simulink model "ups_control_non_linear_load_clean"  (R2024b)
settings: Solver=ode3  StartTime=0.0  StopTime=1  FixedStep=1e-6  MaxStep=1e-6  RelTol=1e-3
libraries: spsParallelRLCBranchLib x9, simulink x4, spsabctodq0Lib x3, eeGeneralControl x3, slpidlib x2, spsUniversalBridgeLib x2, spsGroundLib x2, spsThreePhaseVIMeasurementLib x2, spsDCVoltageSourceLib x1, spsdq0toabcLib x1, spsThreePhaseSeriesRLCBranchLib x1, sps_lib x1
settings Model: Creator=malak  LastModifiedBy=malak

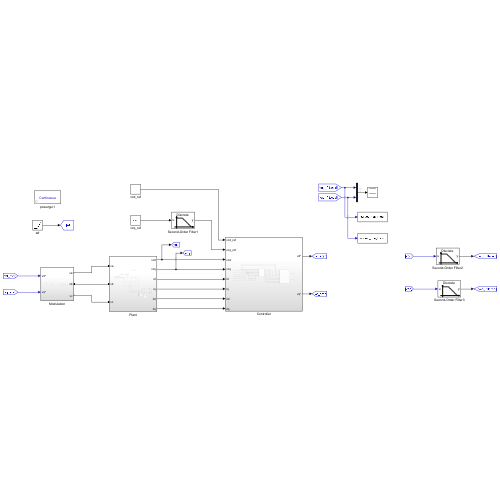
[thumbnail: Simulink's stored preview of the top-level diagram]
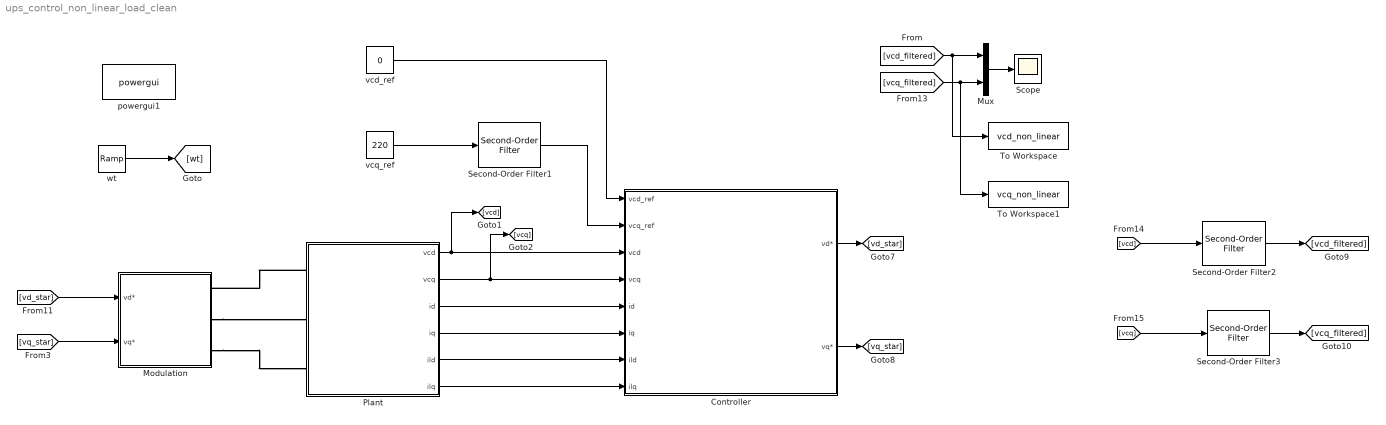
== system ups_control_non_linear_load_clean ==
  Controller : Subsystem
  Modulation : Subsystem
  Mux : Mux  Inputs=2
  Plant : Subsystem
  Scope : Scope
  Second-Order Filter1 : eeGeneralControl/Second-Order Filter  FilterType=Low-pass  fn=60  Zeta=0.707  Ts=-1  A0=0  Ph0=0  f0=0  b0=0
      settings: LibrarySourceBlock=ee_sl_lib/General Control/Second-Order Filter
  Second-Order Filter2 : eeGeneralControl/Second-Order Filter  FilterType=Low-pass  fn=60  Zeta=0.707  Ts=-1  A0=0  Ph0=0  f0=0  b0=0
      settings: LibrarySourceBlock=ee_sl_lib/General Control/Second-Order Filter
  Second-Order Filter3 : eeGeneralControl/Second-Order Filter  FilterType=Low-pass  fn=60  Zeta=0.707  Ts=-1  A0=0  Ph0=0  f0=0  b0=0
      settings: LibrarySourceBlock=ee_sl_lib/General Control/Second-Order Filter
  To Workspace : ToWorkspace  VariableName=vcd_non_linear  SaveFormat=Timeseries  SampleTime=-1
  To Workspace1 : ToWorkspace  VariableName=vcq_non_linear  SaveFormat=Timeseries  SampleTime=-1
  powergui1 : sps_lib/powergui  Priority=1  SimulationMode=Continuous  SampleTime=50e-6  frequency=60  Iterations=50  frequencyindice=0  Pbase=100e6  ErrMax=1e-4  UnitsV=kV  UnitsW=MW  buscounter=0  FunctionMessages=off  echomessages=off  EnableUseOfTLC=off  CurrentSourceSwitches=off  DisableSnubberDevices=off  DisableRonSwitches=off  DisableVfSwitches=off  DisplayEquations=off  AutomaticDiscreteSolvers=off  SolverType=Tustin/Backward Euler (TBE)  Interpol=off  ExternalGateDelay=off  methode=off  Ts=100  x0status=blocks  SPID=on  SwTol=0  HookPort=off  NonlinearTolerance=1e-4  nMaxIteration=100  ContinueOnMaxIteration=off  RestoreLinks=warning  ResistiveCurrentMeasurement=off  Frange=[0:2:500]  Ylog=off  Xlog=on  ShowGrid=off  save=off  variable=ZData  structure=0  ZoomFFT=off  StartTime=0.0  cycles=1  DisplayStyle=1  fundamental=60  FreqAxis=off  MaxFrequency=1000  frequencyindicesteady=1  RmsSteady=1  display=off
  vcd_ref : Constant  Value=0
  vcq_ref : Constant  Value=220
  wt : simulink/Sources/Ramp  slope=2*pi*60  start=0  InitialOutput=0
  wires:
  Second-Order Filter2/1 -> [vcd_filtered]
  [vcd] -> Second-Order Filter2/1
  wt/1 -> [wt]
  Second-Order Filter3/1 -> [vcq_filtered]
  Controller/1(vd*) -> [vd_star]
  [vcq_filtered] -> To Workspace1/1, Mux/2
  vcd_ref/1 -> Controller/1(vcd_ref)
  [vcq] -> Second-Order Filter3/1
  Second-Order Filter1/1 -> Controller/2(vcq_ref)
  Mux/1 -> Scope/1
  vcq_ref/1 -> Second-Order Filter1/1
  [vcd_filtered] -> To Workspace/1, Mux/1
  Controller/2(vq*) -> [vq_star]
  [vq_star] -> Modulation/2(vq*)
  [vd_star] -> Modulation/1(vd*)
  Plant/1(vcd) -> [vcd], Controller/3(vcd)
  Plant/2(vcq) -> [vcq], Controller/4(vcq)
  Plant/3(id) -> Controller/5(id)
  Plant/4(iq) -> Controller/6(iq)
  Plant/5(ild) -> Controller/7(ild)
  Plant/6(ilq) -> Controller/8(ilq)
  connections:
  Plant/LConn1 -- Modulation/RConn1
  Modulation/RConn2 -- Plant/LConn2
  Modulation/RConn3 -- Plant/LConn3

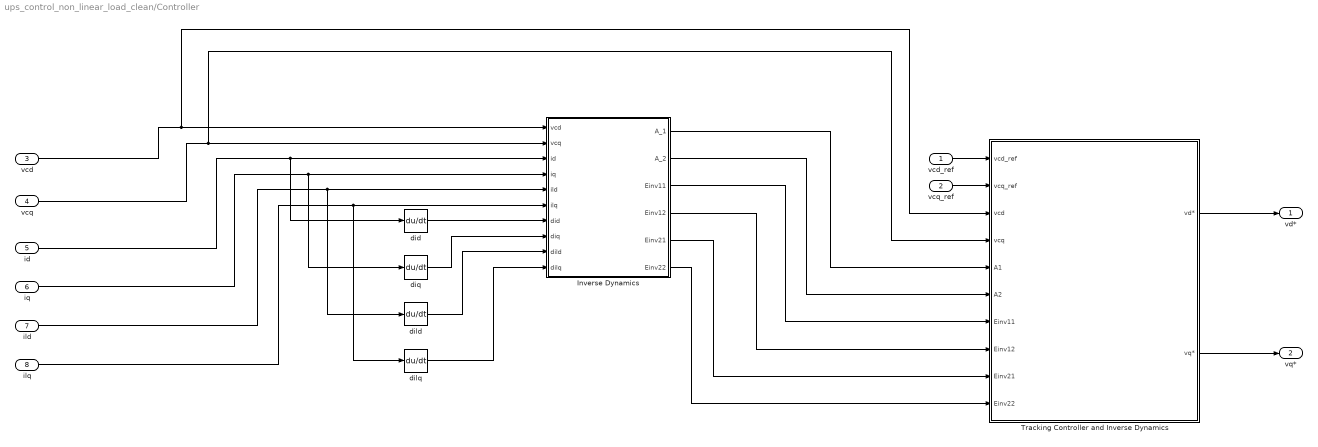
== system ups_control_non_linear_load_clean/Controller ==
  vcd_ref : Inport
  vcq_ref : Inport  Port=2
  vcd : Inport  Port=3
  vcq : Inport  Port=4
  id : Inport  Port=5
  iq : Inport  Port=6
  ild : Inport  Port=7
  ilq : Inport  Port=8
  Inverse Dynamics : MATLAB Function  TreatAsAtomicUnit=on
  Tracking Controller and Inverse Dynamics : Subsystem
  did : Derivative  CoefficientInTFapproximation=500
  dild : Derivative  CoefficientInTFapproximation=500
  dilq : Derivative  CoefficientInTFapproximation=500
  diq : Derivative  CoefficientInTFapproximation=500
  vd* : Outport
  vq* : Outport  Port=2
  wires:
  vcd/1 -> Tracking Controller and Inverse Dynamics/3(vcd), Inverse Dynamics/1(vcd)
  vcq/1 -> Tracking Controller and Inverse Dynamics/4(vcq), Inverse Dynamics/2(vcq)
  id/1 -> did/1, Inverse Dynamics/3(id)
  iq/1 -> diq/1, Inverse Dynamics/4(iq)
  ild/1 -> dild/1, Inverse Dynamics/5(ild)
  ilq/1 -> dilq/1, Inverse Dynamics/6(ilq)
  did/1 -> Inverse Dynamics/7(did)
  diq/1 -> Inverse Dynamics/8(diq)
  dild/1 -> Inverse Dynamics/9(dild)
  dilq/1 -> Inverse Dynamics/10(dilq)
  vcd_ref/1 -> Tracking Controller and Inverse Dynamics/1(vcd_ref)
  vcq_ref/1 -> Tracking Controller and Inverse Dynamics/2(vcq_ref)
  Inverse Dynamics/1(A_1) -> Tracking Controller and Inverse Dynamics/5(A1)
  Inverse Dynamics/2(A_2) -> Tracking Controller and Inverse Dynamics/6(A2)
  Inverse Dynamics/3(Einv11) -> Tracking Controller and Inverse Dynamics/7(Einv11)
  Inverse Dynamics/4(Einv12) -> Tracking Controller and Inverse Dynamics/8(Einv12)
  Inverse Dynamics/5(Einv21) -> Tracking Controller and Inverse Dynamics/9(Einv21)
  Inverse Dynamics/6(Einv22) -> Tracking Controller and Inverse Dynamics/10(Einv22)
  Tracking Controller and Inverse Dynamics/1(vd*) -> vd*/1
  Tracking Controller and Inverse Dynamics/2(vq*) -> vq*/1

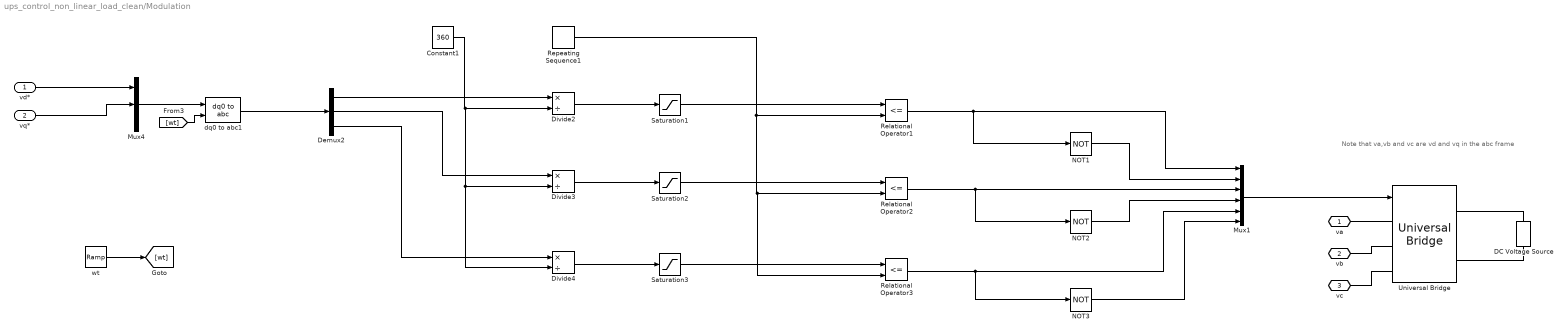
== system ups_control_non_linear_load_clean/Modulation ==
  note: Note that va,vb and vc are vd and vq in the abc frame
  vd* : Inport
  vq* : Inport  Port=2
  Constant1 : Constant  Value=360
  DC Voltage Source : spsDCVoltageSourceLib/DC Voltage Source  Amplitude=360  Measurements=None
  Demux2 : Demux  Outputs=3
  Divide2 : Product  Inputs=*/
  Divide3 : Product  Inputs=*/
  Divide4 : Product  Inputs=*/
  Mux1 : Mux  Inputs=6
  Mux4 : Mux  Inputs=3
  NOT1 : Logic  Operator=NOT  IconShape=distinctive  AllPortsSameDT=off  OutDataTypeStr=boolean
  NOT2 : Logic  Operator=NOT  IconShape=distinctive  AllPortsSameDT=off  OutDataTypeStr=boolean
  NOT3 : Logic  Operator=NOT  IconShape=distinctive  AllPortsSameDT=off  OutDataTypeStr=boolean
  Relational Operator1 : RelationalOperator  Operator=<=  OutDataTypeStr=boolean  RndMeth=Simplest  InputSameDT=off
  Relational Operator2 : RelationalOperator  Operator=<=  OutDataTypeStr=boolean  RndMeth=Simplest  InputSameDT=off
  Relational Operator3 : RelationalOperator  Operator=<=  OutDataTypeStr=boolean  RndMeth=Simplest  InputSameDT=off
  Repeating Sequence1 : simulink/Sources/Repeating Sequence  rep_seq_t=[0 5.5555555555555555555555555555556e-5 1.1111111111111111111111111111111e-4]  rep_seq_y=[-1 +1 -1]
  Saturation1 : Saturate  UpperLimit=1  LowerLimit=-1
  Saturation2 : Saturate  UpperLimit=1  LowerLimit=-1
  Saturation3 : Saturate  UpperLimit=1  LowerLimit=-1
  Universal Bridge : spsUniversalBridgeLib/Universal Bridge  Arms=3  SnubberResistance=1e5  SnubberCapacitance=inf  Device=IGBT / Diodes  Ron=1e-3  Lon=0  ForwardVoltages="[  0  0  ]"  ForwardVoltage=0  GTOparameters=[ 10e-6 , 20e-6 ]  IGBTparameters=[ 1e-6 , 2e-6 ]  Measurements=None  Measurements_2=None  converterType=Rectifier
  dq0 to abc1 : spsdq0toabcLib/dq0 to abc  Alignment=Aligned with phase A axis
  wt : simulink/Sources/Ramp  slope=2*pi*60  start=0  InitialOutput=0
  va : PMIOPort  Side=Right
  vb : PMIOPort  Port=2  Side=Right
  vc : PMIOPort  Port=3  Side=Right
  wires:
  Constant1/1 -> Divide2/2, Divide3/2, Divide4/2
  Mux4/1 -> dq0 to abc1/1
  Saturation1/1 -> Relational Operator1/1
  NOT2/1 -> Mux1/4
  Mux1/1 -> Universal Bridge/1
  vq*/1 -> Mux4/2
  Demux2/2 -> Divide3/1
  NOT3/1 -> Mux1/6
  Saturation2/1 -> Relational Operator2/1
  Relational Operator1/1 -> Mux1/1, NOT1/1
  Relational Operator3/1 -> Mux1/5, NOT3/1
  vd*/1 -> Mux4/1
  Divide2/1 -> Saturation1/1
  Repeating Sequence1/1 -> Relational Operator1/2, Relational Operator2/2, Relational Operator3/2
  Demux2/3 -> Divide4/1
  dq0 to abc1/1 -> Demux2/1
  NOT1/1 -> Mux1/2
  Divide3/1 -> Saturation2/1
  [wt] -> dq0 to abc1/2
  Saturation3/1 -> Relational Operator3/1
  Demux2/1 -> Divide2/1
  Divide4/1 -> Saturation3/1
  Relational Operator2/1 -> Mux1/3, NOT2/1
  wt/1 -> [wt]
  connections:
  Universal Bridge/LConn1 -- va/RConn1
  DC Voltage Source/LConn1 -- Universal Bridge/RConn2
  DC Voltage Source/RConn1 -- Universal Bridge/RConn1
  Universal Bridge/LConn2 -- vb/RConn1
  Universal Bridge/LConn3 -- vc/RConn1

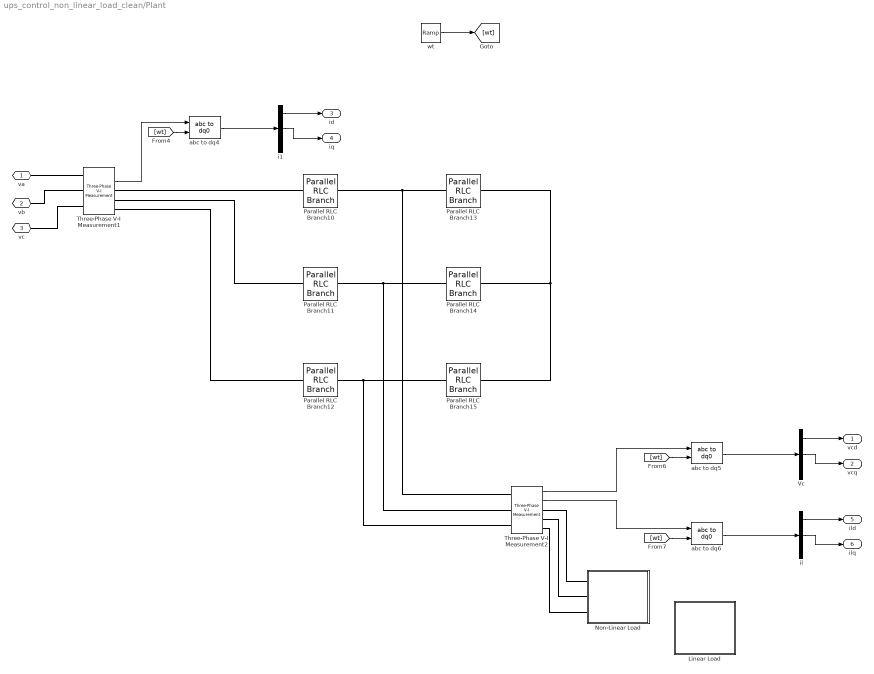
== system ups_control_non_linear_load_clean/Plant ==
  Linear Load : Subsystem
  Non-Linear Load : Subsystem
  Parallel RLC Branch10 : spsParallelRLCBranchLib/Parallel RLC Branch  LConnTagsString=a  RConnTagsString=__new0  BranchType=L  Resistance=10  Inductance=0.000800  SetiL0=off  InitialCurrent=0  Capacitance=0.001650  Setx0=off  InitialVoltage=0  Measurements=None
  Parallel RLC Branch11 : spsParallelRLCBranchLib/Parallel RLC Branch  LConnTagsString=a  RConnTagsString=__new0  BranchType=L  Resistance=10  Inductance=0.000800  SetiL0=off  InitialCurrent=0  Capacitance=0.001650  Setx0=off  InitialVoltage=0  Measurements=None
  Parallel RLC Branch12 : spsParallelRLCBranchLib/Parallel RLC Branch  LConnTagsString=a  RConnTagsString=__new0  BranchType=L  Resistance=10  Inductance=0.000800  SetiL0=off  InitialCurrent=0  Capacitance=0.001650  Setx0=off  InitialVoltage=0  Measurements=None
  Parallel RLC Branch13 : spsParallelRLCBranchLib/Parallel RLC Branch  LConnTagsString=a  RConnTagsString=__new0  BranchType=C  Resistance=10  Inductance=0.000800  SetiL0=off  InitialCurrent=0  Capacitance=0.000075  Setx0=off  InitialVoltage=0  Measurements=None
  Parallel RLC Branch14 : spsParallelRLCBranchLib/Parallel RLC Branch  LConnTagsString=a  RConnTagsString=__new0  BranchType=C  Resistance=10  Inductance=0.000800  SetiL0=off  InitialCurrent=0  Capacitance=0.000075  Setx0=off  InitialVoltage=0  Measurements=None
  Parallel RLC Branch15 : spsParallelRLCBranchLib/Parallel RLC Branch  LConnTagsString=a  RConnTagsString=__new0  BranchType=C  Resistance=10  Inductance=0.000800  SetiL0=off  InitialCurrent=0  Capacitance=0.000075  Setx0=off  InitialVoltage=0  Measurements=None
  Three-Phase V-I Measurement1 : spsThreePhaseVIMeasurementLib/Three-Phase V-I Measurement  VoltageMeasurement=phase-to-ground  SetLabelV=off  LabelV=Vabc  Vpu=off  VpuLL=off  CurrentMeasurement=yes  SetLabelI=off  LabelI=Iabc  Ipu=off  Pbase=100e6  Vbase=500e3  OutputType=Complex  PhasorSimulation=off  PSBequivalent=0
  Three-Phase V-I Measurement2 : spsThreePhaseVIMeasurementLib/Three-Phase V-I Measurement  VoltageMeasurement=phase-to-ground  SetLabelV=off  LabelV=Vabc  Vpu=off  VpuLL=off  CurrentMeasurement=yes  SetLabelI=off  LabelI=Iabc  Ipu=off  Pbase=100e6  Vbase=500e3  OutputType=Complex  PhasorSimulation=off  PSBequivalent=0
  Vc : Demux  Outputs=3
  abc to dq4 : spsabctodq0Lib/abc to dq0  Alignment=Aligned with phase A axis
  abc to dq5 : spsabctodq0Lib/abc to dq0  Alignment=Aligned with phase A axis
  abc to dq6 : spsabctodq0Lib/abc to dq0  Alignment=Aligned with phase A axis
  i1 : Demux  Outputs=3
  il : Demux  Outputs=3
  wt : simulink/Sources/Ramp  slope=2*pi*60  start=0  InitialOutput=0
  va : PMIOPort  Side=Left
  vb : PMIOPort  Port=2  Side=Left
  vc : PMIOPort  Port=3  Side=Left
  vcd : Outport
  vcq : Outport  Port=2
  id : Outport  Port=3
  iq : Outport  Port=4
  ild : Outport  Port=5
  ilq : Outport  Port=6
  wires:
  abc to dq4/1 -> i1/1
  il/1 -> ild/1
  i1/1 -> id/1
  Three-Phase V-I Measurement1/2 -> abc to dq4/1
  il/2 -> ilq/1
  i1/2 -> iq/1
  Vc/2 -> vcq/1
  [wt] -> abc to dq5/2
  Three-Phase V-I Measurement2/1 -> abc to dq5/1
  abc to dq5/1 -> Vc/1
  abc to dq6/1 -> il/1
  [wt] -> abc to dq6/2
  Vc/1 -> vcd/1
  Three-Phase V-I Measurement2/2 -> abc to dq6/1
  [wt] -> abc to dq4/2
  wt/1 -> [wt]
  connections:
  Three-Phase V-I Measurement2/LConn3 -- Parallel RLC Branch12/RConn1 -- Parallel RLC Branch15/LConn1
  Parallel RLC Branch14/RConn1 -- Parallel RLC Branch15/RConn1 -- Parallel RLC Branch13/RConn1
  Three-Phase V-I Measurement2/LConn2 -- Parallel RLC Branch14/LConn1 -- Parallel RLC Branch11/RConn1
  Three-Phase V-I Measurement2/LConn1 -- Parallel RLC Branch13/LConn1 -- Parallel RLC Branch10/RConn1
  Three-Phase V-I Measurement1/RConn3 -- Parallel RLC Branch12/LConn1
  va/RConn1 -- Three-Phase V-I Measurement1/LConn1
  Parallel RLC Branch10/LConn1 -- Three-Phase V-I Measurement1/RConn1
  Three-Phase V-I Measurement1/RConn2 -- Parallel RLC Branch11/LConn1
  vb/RConn1 -- Three-Phase V-I Measurement1/LConn2
  vc/RConn1 -- Three-Phase V-I Measurement1/LConn3
  Non-Linear Load/LConn1 -- Three-Phase V-I Measurement2/RConn1
  Non-Linear Load/LConn2 -- Three-Phase V-I Measurement2/RConn2
  Non-Linear Load/LConn3 -- Three-Phase V-I Measurement2/RConn3

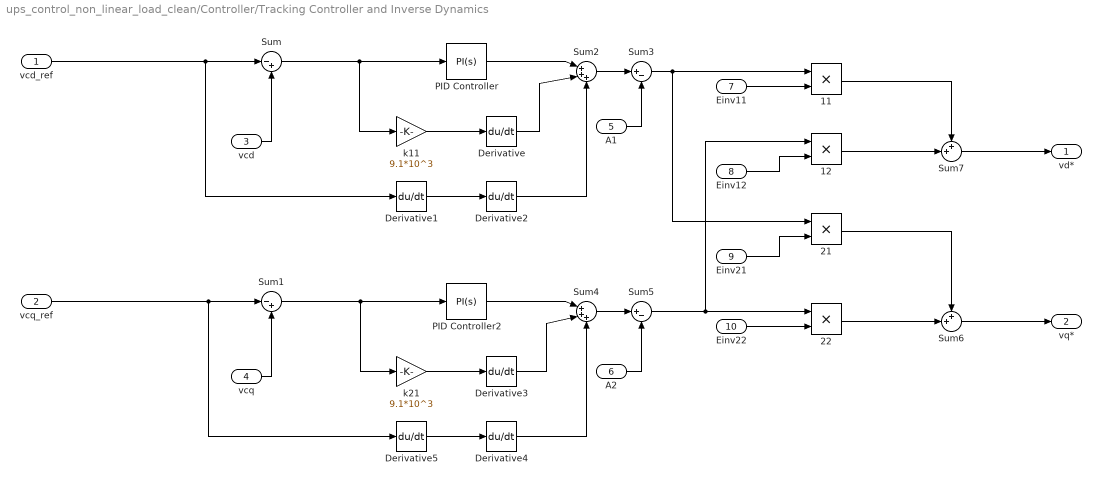
== system ups_control_non_linear_load_clean/Controller/Tracking Controller and Inverse Dynamics ==
  vcd_ref : Inport
  vcq_ref : Inport  Port=2
  vcd : Inport  Port=3
  vcq : Inport  Port=4
  A1 : Inport  Port=5
  A2 : Inport  Port=6
  Einv11 : Inport  Port=7
  Einv12 : Inport  Port=8
  Einv21 : Inport  Port=9
  Einv22 : Inport  Port=10
  {11..12,21..22} (4 alike) : Product
  Derivative{,1..5} (6 alike) : Derivative  CoefficientInTFapproximation=500
  PID Controller : slpidlib/PID Controller  Controller=PI  Form=Parallel  TimeDomain=Continuous-time  UseExternalTs=off  SampleTime=-1  IntegratorMethod=Forward Euler  FilterMethod=Forward Euler  ControllerParametersSource=internal  P=2.115*10^7  I=2.025*10^9  UseKiTs=off  D=0  UseExternalDerivativeSource=off  N=100  UseFilter=on  TunerSelectOption=Transfer Function Based (PID Tuner App)  InitialConditionSource=internal  InitialConditionForIntegrator=0  InitialConditionForFilter=0  DifferentiatorICPrevScaledInput=0  ExternalReset=none  TrackingMode=off  Kt=1  LimitOutput=off  SatLimitsSource=internal  UpperSaturationLimit=inf  LowerSaturationLimit=-inf  LinearizeAsGain=on  AntiWindupMode=none  Kb=1  LimitIntegrator=off  UpperIntegratorSaturationLimit=inf  LowerIntegratorSaturationLimit=-inf  POutMin=[]  POutMax=[]  IOutMin=[]  IOutMax=[]  DOutMin=[]  DOutMax=[]  NOutMin=[]  NOutMax=[]  SumOutMin=[]  SumOutMax=[]  SaturationOutMin=[]  SaturationOutMax=[]  PParamMin=[]  PParamMax=[]  IParamMin=[]  IParamMax=[]  DParamMin=[]  DParamMax=[]  NParamMin=[]  NParamMax=[]  KbParamMin=[]  KbParamMax=[]  KtParamMin=[]  KtParamMax=[]  KbOutMin=[]  KbOutMax=[]  KtOutMin=[]  KtOutMax=[]  IntegratorOutMin=[]  IntegratorOutMax=[]  FilterOutMin=[]  FilterOutMax=[]  SumI1OutMin=[]  SumI1OutMax=[]  SumI2OutMin=[]  SumI2OutMax=[]  SumI3OutMin=[]  SumI3OutMax=[]  SumI4OutMin=[]  SumI4OutMax=[]  SumDOutMin=[]  SumDOutMax=[]  DifferentiatorOutMin=[]  DifferentiatorOutMax=[]  FilterDiffOutCoefMin=[]  FilterDiffOutCoefMax=[]  ReciprocalOutMin=[]  ReciprocalOutMax=[]  SumDenOutMin=[]  SumDenOutMax=[]  SumNumOutMin=[]  SumNumOutMax=[]  DivideOutMin=[]  DivideOutMax=[]  UdiffTsProdOutMin=[]  UdiffTsProdOutMax=[]  NTsProdOutMin=[]  NTsProdOutMax=[]  UintegralTsProdOutMin=[]  UintegralTsProdOutMax=[]  UngainTsProdOutMin=[]  UngainTsProdOutMax=[]  ClampingZeroOutDataTypeStr=Inherit: Inherit via back propagation  ClampingZeroOutMin=[]  ClampingZeroOutMax=[]  FilterDenConstantOutDataTypeStr=Inherit: Inherit via back propagation  FilterDenConstantOutMin=[]  FilterDenConstantOutMax=[]  PCopyOutDataTypeStr=Inherit: Inherit via back propagation  PCopyOutMin=[]  PCopyOutMax=[]  NCopyOutDataTypeStr=Inherit: Inherit via back propagation  NCopyOutMin=[]  NCopyOutMax=[]  IntegratorContinuousStateAttributes=''  IntegratorStateMustResolveToSignalObject=off  IntegratorRTWStateStorageClass=Auto  FilterContinuousStateAttributes=''  FilterStateMustResolveToSignalObject=off  FilterRTWStateStorageClass=Auto  ParallelPVariant=InternalParameters  IdealPVariant=Disabled  IVariant=InternalParameters  DVariant=Disabled  IntegratorVariant=Continuous  SatVariant=Disabled  AWVariant=Passthrough  PCopyVariant=Disabled  TRVariant=Disabled  FdbkBlocksVariant=Forward  IdealPFdbkVariant=Disabled  SatFdbkVariant=Disabled  DerivativeFilterVariant=Disabled  NVariant=Disabled  NCopyVariant=Disabled_SignalSpec  FilterICVariant=Disabled  IntegratorICVariant=InternalICs  ExternalResetVariant=Disabled  TRSumVariant=Passthrough  SumFdbkVariant=Disabled  SumVariant=Sum_PI  TsampFilterVariant=InternalTs  TsampNgainVariant=Passthrough  TsampIntegralVariant=Disabled_SignalSpec  ExternalSaturationOutDataTypeStr=Inherit: Same as second input  DerivativeSourceVariant=Disabled  PreIntVariant=InternalPreInt
  PID Controller2 : slpidlib/PID Controller  Controller=PI  Form=Parallel  TimeDomain=Continuous-time  UseExternalTs=off  SampleTime=-1  IntegratorMethod=Forward Euler  FilterMethod=Forward Euler  ControllerParametersSource=internal  P=2.115*10^7  I=2.025*10^9  UseKiTs=off  D=0  UseExternalDerivativeSource=off  N=100  UseFilter=on  TunerSelectOption=Transfer Function Based (PID Tuner App)  InitialConditionSource=internal  InitialConditionForIntegrator=0  InitialConditionForFilter=0  DifferentiatorICPrevScaledInput=0  ExternalReset=none  TrackingMode=off  Kt=1  LimitOutput=off  SatLimitsSource=internal  UpperSaturationLimit=inf  LowerSaturationLimit=-inf  LinearizeAsGain=on  AntiWindupMode=none  Kb=1  LimitIntegrator=off  UpperIntegratorSaturationLimit=inf  LowerIntegratorSaturationLimit=-inf  POutMin=[]  POutMax=[]  IOutMin=[]  IOutMax=[]  DOutMin=[]  DOutMax=[]  NOutMin=[]  NOutMax=[]  SumOutMin=[]  SumOutMax=[]  SaturationOutMin=[]  SaturationOutMax=[]  PParamMin=[]  PParamMax=[]  IParamMin=[]  IParamMax=[]  DParamMin=[]  DParamMax=[]  NParamMin=[]  NParamMax=[]  KbParamMin=[]  KbParamMax=[]  KtParamMin=[]  KtParamMax=[]  KbOutMin=[]  KbOutMax=[]  KtOutMin=[]  KtOutMax=[]  IntegratorOutMin=[]  IntegratorOutMax=[]  FilterOutMin=[]  FilterOutMax=[]  SumI1OutMin=[]  SumI1OutMax=[]  SumI2OutMin=[]  SumI2OutMax=[]  SumI3OutMin=[]  SumI3OutMax=[]  SumI4OutMin=[]  SumI4OutMax=[]  SumDOutMin=[]  SumDOutMax=[]  DifferentiatorOutMin=[]  DifferentiatorOutMax=[]  FilterDiffOutCoefMin=[]  FilterDiffOutCoefMax=[]  ReciprocalOutMin=[]  ReciprocalOutMax=[]  SumDenOutMin=[]  SumDenOutMax=[]  SumNumOutMin=[]  SumNumOutMax=[]  DivideOutMin=[]  DivideOutMax=[]  UdiffTsProdOutMin=[]  UdiffTsProdOutMax=[]  NTsProdOutMin=[]  NTsProdOutMax=[]  UintegralTsProdOutMin=[]  UintegralTsProdOutMax=[]  UngainTsProdOutMin=[]  UngainTsProdOutMax=[]  ClampingZeroOutDataTypeStr=Inherit: Inherit via back propagation  ClampingZeroOutMin=[]  ClampingZeroOutMax=[]  FilterDenConstantOutDataTypeStr=Inherit: Inherit via back propagation  FilterDenConstantOutMin=[]  FilterDenConstantOutMax=[]  PCopyOutDataTypeStr=Inherit: Inherit via back propagation  PCopyOutMin=[]  PCopyOutMax=[]  NCopyOutDataTypeStr=Inherit: Inherit via back propagation  NCopyOutMin=[]  NCopyOutMax=[]  IntegratorContinuousStateAttributes=''  IntegratorStateMustResolveToSignalObject=off  IntegratorRTWStateStorageClass=Auto  FilterContinuousStateAttributes=''  FilterStateMustResolveToSignalObject=off  FilterRTWStateStorageClass=Auto  ParallelPVariant=InternalParameters  IdealPVariant=Disabled  IVariant=InternalParameters  DVariant=Disabled  IntegratorVariant=Continuous  SatVariant=Disabled  AWVariant=Passthrough  PCopyVariant=Disabled  TRVariant=Disabled  FdbkBlocksVariant=Forward  IdealPFdbkVariant=Disabled  SatFdbkVariant=Disabled  DerivativeFilterVariant=Disabled  NVariant=Disabled  NCopyVariant=Disabled_SignalSpec  FilterICVariant=Disabled  IntegratorICVariant=InternalICs  ExternalResetVariant=Disabled  TRSumVariant=Passthrough  SumFdbkVariant=Disabled  SumVariant=Sum_PI  TsampFilterVariant=InternalTs  TsampNgainVariant=Passthrough  TsampIntegralVariant=Disabled_SignalSpec  ExternalSaturationOutDataTypeStr=Inherit: Same as second input  DerivativeSourceVariant=Disabled  PreIntVariant=InternalPreInt
  Sum : Sum  Inputs=|-+
  Sum1 : Sum  Inputs=|-+
  Sum2 : Sum  Inputs=|+++
  Sum3 : Sum  Inputs=|+-
  Sum4 : Sum  Inputs=|+++
  Sum5 : Sum  Inputs=|+-
  Sum6 : Sum  Inputs=++|
  Sum7 : Sum  Inputs=++|
  k11 : Gain  Gain=9.1*10^3
  k21 : Gain  Gain=9.1*10^3
  vd* : Outport
  vq* : Outport  Port=2
  wires:
  Sum2/1 -> Sum3/1
  Sum4/1 -> Sum5/1
  Derivative/1 -> Sum2/2
  Sum1/1 -> k21/1, PID Controller2/1
  vcd_ref/1 -> Sum/1, Derivative1/1
  PID Controller2/1 -> Sum4/1
  PID Controller/1 -> Sum2/1
  22/1 -> Sum6/2
  21/1 -> Sum6/1
  11/1 -> Sum7/1
  Sum5/1 -> 12/1, 22/1
  Derivative2/1 -> Sum2/3
  12/1 -> Sum7/2
  Sum3/1 -> 11/1, 21/1
  Derivative3/1 -> Sum4/2
  Sum/1 -> k11/1, PID Controller/1
  k11/1 -> Derivative/1
  Derivative1/1 -> Derivative2/1
  vcd/1 -> Sum/2
  vcq_ref/1 -> Derivative5/1, Sum1/1
  vcq/1 -> Sum1/2
  k21/1 -> Derivative3/1
  Derivative5/1 -> Derivative4/1
  Derivative4/1 -> Sum4/3
  A1/1 -> Sum3/2
  A2/1 -> Sum5/2
  Einv11/1 -> 11/2
  Einv12/1 -> 12/2
  Einv21/1 -> 21/2
  Einv22/1 -> 22/2
  Sum6/1 -> vq*/1
  Sum7/1 -> vd*/1

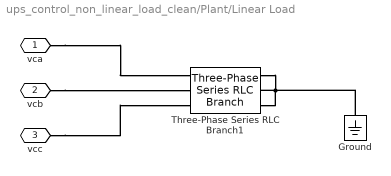
== system ups_control_non_linear_load_clean/Plant/Linear Load ==
  Ground : spsGroundLib/Ground  LConnTagsString=a
  Three-Phase Series RLC Branch1 : spsThreePhaseSeriesRLCBranchLib/Three-Phase Series RLC Branch  LConnTagsString=A|B|C  RConnTagsString=A|B|C  BranchType=RL  Resistance=10  Inductance=0.0035  Capacitance=1e-6  Measurements=None
  vca : PMIOPort  Side=Left
  vcb : PMIOPort  Port=2  Side=Left
  vcc : PMIOPort  Port=3  Side=Left
  connections:
  Ground/LConn1 -- Three-Phase Series RLC Branch1/RConn2 -- Three-Phase Series RLC Branch1/RConn3 -- Three-Phase Series RLC Branch1/RConn1
  vcb/RConn1 -- Three-Phase Series RLC Branch1/LConn2
  vcc/RConn1 -- Three-Phase Series RLC Branch1/LConn3
  vca/RConn1 -- Three-Phase Series RLC Branch1/LConn1

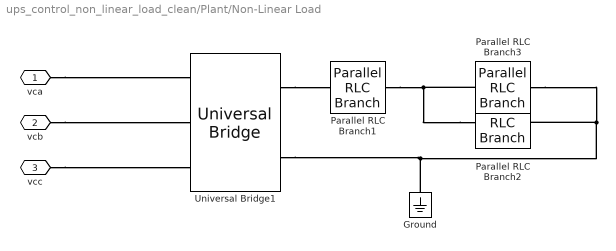
== system ups_control_non_linear_load_clean/Plant/Non-Linear Load ==
  Ground : spsGroundLib/Ground  LConnTagsString=a
  Parallel RLC Branch1 : spsParallelRLCBranchLib/Parallel RLC Branch  LConnTagsString=a  RConnTagsString=__new0  BranchType=L  Resistance=10  Inductance=0.0047  SetiL0=off  InitialCurrent=0  Capacitance=0.001650  Setx0=off  InitialVoltage=0  Measurements=None
  Parallel RLC Branch2 : spsParallelRLCBranchLib/Parallel RLC Branch  LConnTagsString=a  RConnTagsString=__new0  BranchType=R  Resistance=40  Inductance=0.000800  SetiL0=off  InitialCurrent=0  Capacitance=0.000075  Setx0=off  InitialVoltage=0  Measurements=None
  Parallel RLC Branch3 : spsParallelRLCBranchLib/Parallel RLC Branch  LConnTagsString=a  RConnTagsString=__new0  BranchType=C  Resistance=10  Inductance=0.000800  SetiL0=off  InitialCurrent=0  Capacitance=0.001650  Setx0=off  InitialVoltage=0  Measurements=None
  Universal Bridge1 : spsUniversalBridgeLib/Universal Bridge  Arms=3  SnubberResistance=1e5  SnubberCapacitance=inf  Device=Diodes  Ron=1e-3  Lon=0  ForwardVoltages="[  0  0  ]"  ForwardVoltage=0  GTOparameters=[ 10e-6 , 20e-6 ]  IGBTparameters=[ 1e-6 , 2e-6 ]  Measurements=None  Measurements_2=None  converterType=Rectifier
  vca : PMIOPort  Side=Left
  vcb : PMIOPort  Port=2  Side=Left
  vcc : PMIOPort  Port=3  Side=Left
  connections:
  vcb/RConn1 -- Universal Bridge1/LConn2
  vcc/RConn1 -- Universal Bridge1/LConn3
  vca/RConn1 -- Universal Bridge1/LConn1
  Universal Bridge1/RConn1 -- Parallel RLC Branch1/LConn1
  Parallel RLC Branch2/LConn1 -- Parallel RLC Branch3/LConn1 -- Parallel RLC Branch1/RConn1
  Parallel RLC Branch2/RConn1 -- Parallel RLC Branch3/RConn1 -- Ground/LConn1 -- Universal Bridge1/RConn2

== matlab function ups_control_non_linear_load_clean/Controller/Inverse Dynamics ==
  data: vcd input; vcq input; A_1 output; A_2 output; id input; iq input; ild input; ilq input; did input; diq input; dild input; Einv11 output; dilq input; Einv12 output; Einv21 output; Einv22 output
function [A_1,A_2,Einv11,Einv12,Einv21,Einv22] = Inverse_Dynamics(vcd,vcq,id,iq,ild,ilq,did,diq,dild,dilq)
w = 60;
C_f = 0.000075;
L_f = 0.0008;




p = vcd*ild+vcq*ilq; % calculating real power
q = vcq*ild - vcd*ilq - w*C_f*(vcq^2+vcd^2) + w*L_f*(iq^2+id^2); % calculating imaginary power


denom=C_f*(vcd^2+vcq^2);


dvcd = id/C_f - p*vcd/denom - (q-w*L_f*(id^2+iq^2))*vcq/denom; % calculting derivative of vcd
dvcq = iq/C_f - p*vcq/denom + (q-w*L_f*(id^2+iq^2))*vcd/denom; % calculting derivative of vcq

%did = w*iq-vcd/L_f + vd/L_f;

%diq = -w*id-vcq/L_f + vq/L_f;


p_dot = dvcd*ild + vcd*dild + dvcq*ilq +vcq*dilq;

q_dot = dvcq*ild + vcq*dild - dvcd*ilq - vcd*dilq ...
    - 2*w*C_f*(vcq*dvcq+vcd*dvcd) + 2*w*L_f*(iq*diq + id*did);
%p_dot=dvcd*ild+dild*vcd+dvcq*ilq+vcq*dilq;
%q_dot=dvcd*ild+dild*vcd-dvcq*ilq-vcq*dilq-2*60*0.000075*(vcq*dvcq+vcd*dvcd)+2*60*0.0008*(ilq+ild)*(dilq+dild);
x1 = id;
x2 = iq;
x3 = vcd;
x4 = vcq;

V = x3^2 + x4^2;
I = x1^2+x2^2;






A_1 = (w/C_f)*x2-(1/(L_f*C_f))*x3-p*x1/((C_f^2)*V)-p_dot*x3/(C_f*V)-q_dot*x4/(C_f*V)...
    -(q-w*L_f*I)*x2/(C_f*C_f*V)-((q-w*L_f*I)^2)*x3/((C_f*V)^2)-2*w*(x1*x3+x2*x4)*x4/(C_f*V)...
    -p*(p-2*(x1*x3+x2*x4))*x3/((C_f*V)^2)+2*(q-w*L_f*I)*(x1*x3+x2*x4)*x4/((C_f*V)^2);


A_2 = -(w/C_f)*x1-(1/(L_f*C_f))*x4-p*x2/((C_f^2)*V)-p_dot*x4/(C_f*V)+q_dot*x3/(C_f*V)...
    +(q-w*L_f*I)*x1/(C_f*C_f*V)-((q-w*L_f*I)^2)*x4/((C_f*V)^2)+2*w*(x1*x3+x2*x4)*x3/(C_f*V)...
    -p*(p-2*(x1*x3+x2*x4))*x4/((C_f*V)^2)-2*(q-w*L_f*I)*(x1*x3+x2*x4)*x3/((C_f*V)^2);



% calculating the inverse of the decoupling matrix
Einv11=L_f*C_f*(V-2*w*L_f*x2*x3)/(V+2*w*L_f*(x1*x4-x2*x3));  

Einv12=(-2*w*((L_f)^2)*C_f*x2*x4)/(V+2*w*L_f*(x1*x4-x2*x3));

Einv21=(2*w*((L_f)^2)*C_f*x1*x3)/(V+2*w*L_f*(x1*x4-x2*x3));

Einv22=L_f*C_f*(V+2*w*L_f*x1*x4)/(V+2*w*L_f*(x1*x4-x2*x3));


end
